simulink model "ref_complesso"  (R2023b)
settings: Solver=VariableStepAuto  StartTime=0.0  StopTime=f_lin_RLS_step4_4sin20_05_5sin20_4step_3_2(1, end)  RelTol=1e-3
settings Model: Creator=lollo  LastModifiedBy=lollo

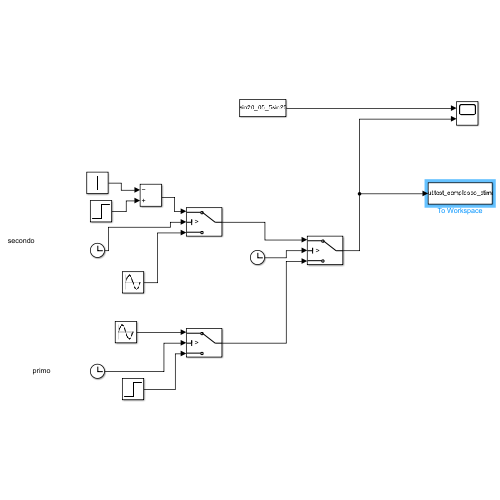
[thumbnail: Simulink's stored preview of the top-level diagram]
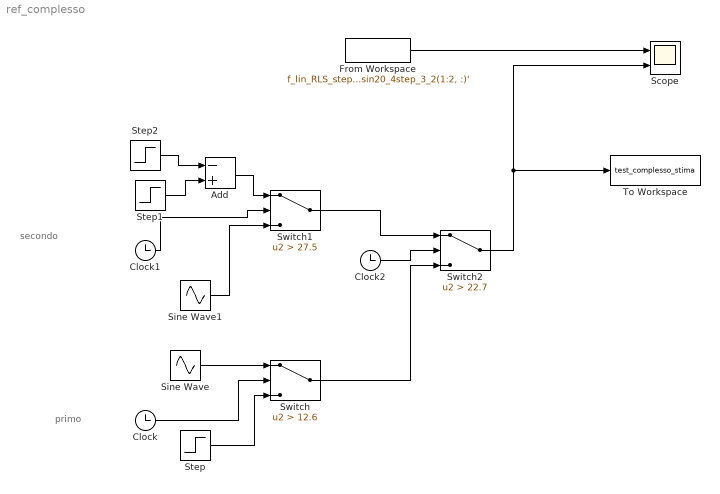
== system ref_complesso ==
  note: secondo
  note: primo
  Add : Sum  Inputs=-+
  Clock : Clock
  Clock1 : Clock
  Clock2 : Clock
  From Workspace : FromWorkspace  VariableName=f_lin_RLS_step4_4sin20_05_5sin20_4step_3_2(1:2, :)'  SampleTime=0.002
  Scope : Scope  NumInputPorts=2
  Sine Wave : Sin  Amplitude=0.0005  Bias=0.004  Frequency=20  SampleTime=0
  Sine Wave1 : Sin  Amplitude=0.0005  Bias=0.005  Frequency=20  SampleTime=0
  Step : Step  Time=2  After=0.004  SampleTime=0
  Step1 : Step  Time=2  After=0.004  SampleTime=0
  Step2 : Step  Time=35.2  After=0.001  SampleTime=0
  Switch : Switch  Criteria=u2 > Threshold  Threshold=12.6  SaturateOnIntegerOverflow=off  InputSameDT=off
  Switch1 : Switch  Criteria=u2 > Threshold  Threshold=27.5  SaturateOnIntegerOverflow=off  InputSameDT=off
  Switch2 : Switch  Criteria=u2 > Threshold  Threshold=22.7  SaturateOnIntegerOverflow=off  InputSameDT=off
  To Workspace : ToWorkspace  VariableName=test_complesso_stima  SampleTime=-1
  wires:
  From Workspace/1 -> Scope/1
  Switch2/1 -> To Workspace/1, Scope/2
  Clock2/1 -> Switch2/2
  Switch/1 -> Switch2/3
  Sine Wave/1 -> Switch/1
  Clock/1 -> Switch/2
  Step/1 -> Switch/3
  Clock1/1 -> Switch1/2
  Sine Wave1/1 -> Switch1/3
  Step1/1 -> Add/2
  Switch1/1 -> Switch2/1
  Add/1 -> Switch1/1
  Step2/1 -> Add/1
